simulink model "Isentity_Model"  (R2024b)
settings: Solver=VariableStepAuto  StartTime=0.0  StopTime=10.0  RelTol=1e-3
libraries: NSA_DEVS_SINKS x3, NSA_DEVS_LOGISTICS x2, NSA_DEVS_SOURCES x2, NSA_DEVS_ROUTING x1
settings Model: Creator=david  LastModifiedBy=peter
settings RTWCC: GPUComputeCapability=3.5

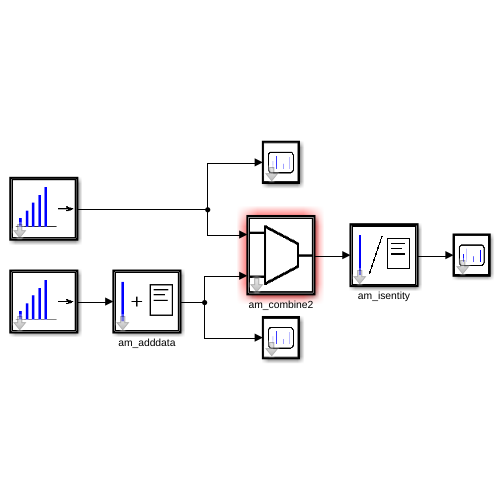
[thumbnail: Simulink's stored preview of the top-level diagram]
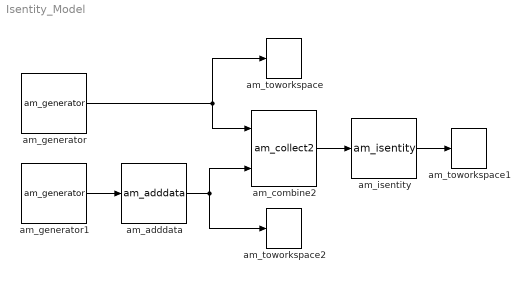
== system Isentity_Model ==
  am_adddata : NSA_DEVS_LOGISTICS/am_adddata  fields="[\"age\"]"  values=[42]  numeric=[true]  infield="\"id\""  tau=[0,1]  debug=0
      settings: SourceProductName=Logistics
  am_combine2 : NSA_DEVS_ROUTING/am_collect2  tD=[0,2]  tau=[0,1]  debug=0
      settings: SourceProductName=Routing
  am_generator : NSA_DEVS_SOURCES/am_generator  tG=5  n0=5  nG=2  tD=[0,2]  debug=0
      settings: SourceProductName=Sources
  am_generator1 : NSA_DEVS_SOURCES/am_generator  tG=1  n0=1  nG=4  tD=[0,2]  debug=0
      settings: SourceProductName=Sources
  am_isentity : NSA_DEVS_LOGISTICS/am_isentity  tau=[0,1]  debug=0
      settings: SourceProductName=Logistics
  am_toworkspace : NSA_DEVS_SINKS/am_toworkspace  varname="\"inVal\""  t0=0  format="\"vector\""  tau=[0,5]  debug=0
      settings: SourceProductName=Sinks
  am_toworkspace1 : NSA_DEVS_SINKS/am_toworkspace  varname="\"Out\""  t0=0  format="\"vector\""  tau=[0,5]  debug=0
      settings: SourceProductName=Sinks
  am_toworkspace2 : NSA_DEVS_SINKS/am_toworkspace  varname="\"inEnt\""  t0=0  format="\"vector\""  tau=[0,5]  debug=0
      settings: SourceProductName=Sinks
  wires:
  am_isentity/1 -> am_toworkspace1/1
  am_combine2/1 -> am_isentity/1
  am_generator/1 -> am_combine2/1, am_toworkspace/1
  am_generator1/1 -> am_adddata/1
  am_adddata/1 -> am_combine2/2, am_toworkspace2/1
